simulink model "chap11_4sim"  (Simulink 7.7)
settings: Solver=ode45  StartTime=0.0  StopTime=10.0  RelTol=1e-3
settings Model: Creator=ljk  LastModifiedBy=ljk  ExtModeTrigMode=oneshot  ExtModeArmWhenConnect=off
settings DataIOCC: LimitDataPoints=off
settings OptimizationCC: BlockReduction=off  BooleanDataType=off
settings DebuggingCC: SaveWithParameterizedLinksMsg=none  SignalResolutionControl=TryResolveAllWithWarning  SolverPrmCheckMsg=none  MultiTaskDSMMsg=warning  MultiTaskCondExecSysMsg=none  StrictBusMsg=None
settings HardwareCC: TargetUnknown=on
settings RTWCC: IncludeERTFirstTime=on

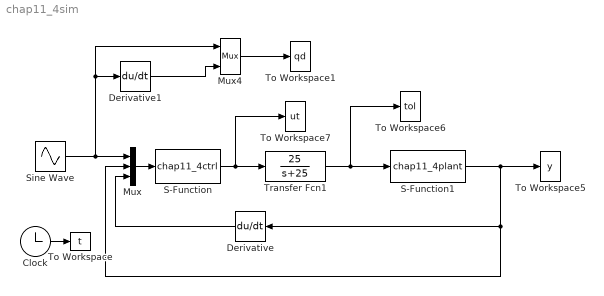
== system chap11_4sim ==
  Clock : Clock
  Derivative : Derivative
  Derivative1 : Derivative
  Mux : Mux  Inputs=3
  Mux4 : Mux  Inputs=2
  S-Function : S-Function  FunctionName=chap11_4ctrl  EnableBusSupport=off
  S-Function1 : S-Function  FunctionName=chap11_4plant  EnableBusSupport=off
  Sine Wave : Sin  Frequency=2*pi  SampleTime=0
  To Workspace : ToWorkspace  VariableName=t  SampleTime=-1  SaveFormat=Array
  To Workspace1 : ToWorkspace  VariableName=qd  SampleTime=-1  SaveFormat=Array
  To Workspace5 : ToWorkspace  VariableName=y  SampleTime=-1  SaveFormat=Array
  To Workspace6 : ToWorkspace  VariableName=tol  SampleTime=-1  SaveFormat=Array
  To Workspace7 : ToWorkspace  VariableName=ut  SampleTime=-1  SaveFormat=Array
  Transfer Fcn1 : TransferFcn  Numerator=[25]  Denominator=[1 25]
  wires:
  Mux/1 -> S-Function/1
  Derivative/1 -> Mux/3
  Sine Wave/1 -> Mux/1, Mux4/1, Derivative1/1
  S-Function1/1 -> Derivative/1, Mux/2, To Workspace5/1
  S-Function/1 -> To Workspace7/1, Transfer Fcn1/1
  Clock/1 -> To Workspace/1
  Transfer Fcn1/1 -> S-Function1/1, To Workspace6/1
  Derivative1/1 -> Mux4/2
  Mux4/1 -> To Workspace1/1
